simulink model "Simulink_Modell"  (R2017b)
settings: Solver=VariableStepAuto  StartTime=0.0  StopTime=10.0  RelTol=1e-3
libraries: simulink x3, aerolibatmos2 x1
settings Model: Creator=Christian Re  LastModifiedBy=Christian Re

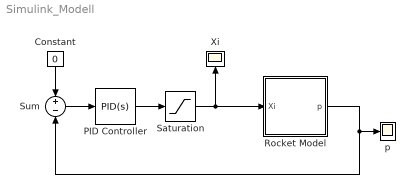
== system Simulink_Modell ==
  Constant : Constant  Value=0
  PID Controller : simulink/Continuous/PID Controller  Controller=PID  TimeDomain=Continuous-time  SampleTime=-1  IntegratorMethod=Forward Euler  FilterMethod=Forward Euler  Form=Parallel  UseFilter=on  ControllerParametersSource=internal  P=0.005  I=0.005  D=0.00008  N=100  InitialConditionSource=internal  InitialConditionForIntegrator=0  InitialConditionForFilter=0  ExternalReset=none  LimitOutput=off  UpperSaturationLimit=inf  LowerSaturationLimit=-inf  LinearizeAsGain=on  AntiWindupMode=none  Kb=1  TrackingMode=off  Kt=1  PParamMin=[]  PParamMax=[]  IParamMin=[]  IParamMax=[]  DParamMin=[]  DParamMax=[]  NParamMin=[]  NParamMax=[]  KbParamMin=[]  KbParamMax=[]  KtParamMin=[]  KtParamMax=[]  POutMin=[]  POutMax=[]  IOutMin=[]  IOutMax=[]  DOutMin=[]  DOutMax=[]  NOutMin=[]  NOutMax=[]  KbOutMin=[]  KbOutMax=[]  KtOutMin=[]  KtOutMax=[]  IntegratorOutMin=[]  IntegratorOutMax=[]  FilterOutMin=[]  FilterOutMax=[]  SumOutMin=[]  SumOutMax=[]  SumI1OutMin=[]  SumI1OutMax=[]  SumI2OutMin=[]  SumI2OutMax=[]  SumI3OutMin=[]  SumI3OutMax=[]  SumDOutMin=[]  SumDOutMax=[]  SaturationOutMin=[]  SaturationOutMax=[]  IntegratorContinuousStateAttributes=''  IntegratorStateMustResolveToSignalObject=off  IntegratorRTWStateStorageClass=Auto  FilterContinuousStateAttributes=''  FilterStateMustResolveToSignalObject=off  FilterRTWStateStorageClass=Auto  DifferentiatorICPrevScaledInput=0  DifferentiatorOutMin=[]  DifferentiatorOutMax=[]  InitialConditionSetting=State (most efficient)  FilterDiffOutCoefMin=[]  FilterDiffOutCoefMax=[]  SumDenOutMin=[]  SumDenOutMax=[]  SumNumOutMin=[]  SumNumOutMax=[]  ReciprocalOutMin=[]  ReciprocalOutMax=[]  DivideOutMin=[]  DivideOutMax=[]  TunerSelectOption=Frequency Response Based
  "Rocket Model " : Subsystem  TreatAsAtomicUnit=on
  Saturation : Saturate  UpperLimit=pi/4  LowerLimit=-pi/4
  Sum : Sum  Inputs=+-
  Xi : Scope
  p : Scope
  wires:
  Sum/1 -> PID Controller/1
  Constant/1 -> Sum/1
  "Rocket Model "/1(p) -> Sum/2, p/1
  PID Controller/1 -> Saturation/1
  Saturation/1 -> "Rocket Model "/1(Xi), Xi/1

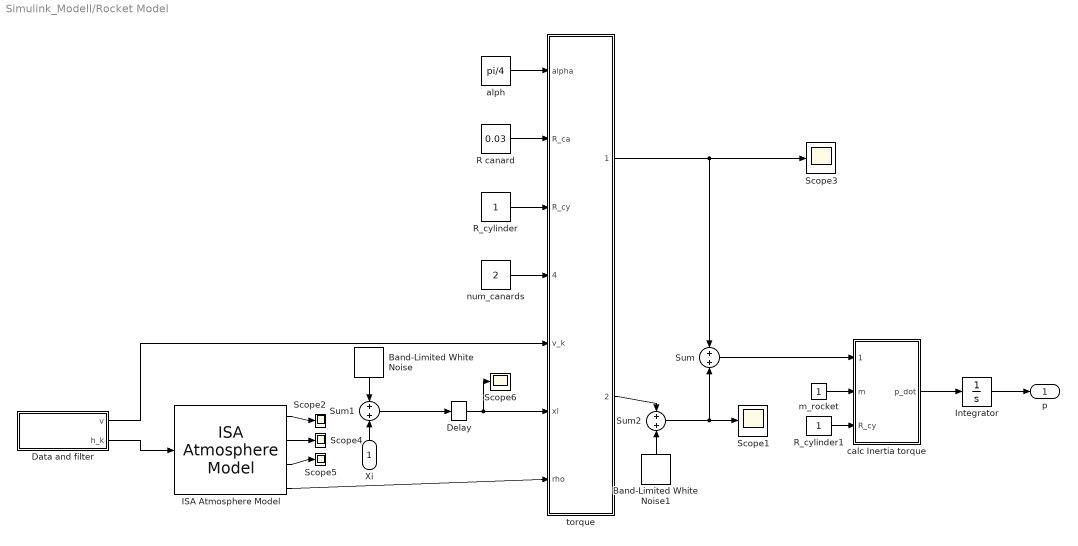
== system Simulink_Modell/Rocket Model  ==
  Xi : Inport
  Band-Limited White Noise : simulink/Sources/Band-Limited White Noise  Cov=[0.0000]  Ts=0.1  seed=[23341]
  Band-Limited White Noise1 : simulink/Sources/Band-Limited White Noise  Cov=[0.0]  Ts=0.1  seed=[23341]
  Data and filter : Subsystem  TreatAsAtomicUnit=on
  Delay : TransportDelay  DelayTime=0.00
  ISA Atmosphere Model : aerolibatmos2/ISA Atmosphere Model  custom=off  g=9.80665  gamma=1.4  R=287.0531  L=0.0065  h_trop=11000  h_strat=20000  rho0=1.225  P0=101325  T0=288.15  h0=0
      settings: SourceProductName=Aerospace Blockset
  Integrator : Integrator
  R canard : Constant  Value=0.03
  R_cylinder : Constant
  R_cylinder1 : Constant
  Scope{1..6} (6 alike) : Scope
  Sum : Sum
  Sum1 : Sum
  Sum2 : Sum
  "alph " : Constant  Value=pi/4
  calc Inertia torque : MATLAB Function  TreatAsAtomicUnit=on
  m_rocket : Constant
  "num_canards " : Constant  Value=2
  torque : MATLAB Function  TreatAsAtomicUnit=on
  p : Outport
  wires:
  "alph "/1 -> torque/1(alpha)
  R canard/1 -> torque/2(R_ca)
  Data and filter/1(v) -> torque/5(v_k)
  "num_canards "/1 -> torque/4(num_c)
  R_cylinder/1 -> torque/3(R_cy)
  m_rocket/1 -> calc Inertia torque/2(m)
  torque/1(M_canard) -> Scope3/1, Sum/1
  Sum/1 -> calc Inertia torque/1(M_sum)
  calc Inertia torque/1(p_dot) -> Integrator/1
  Integrator/1 -> p/1
  R_cylinder1/1 -> calc Inertia torque/3(R_cy)
  Band-Limited White Noise/1 -> Sum1/1
  Xi/1 -> Sum1/2
  Sum1/1 -> Delay/1
  Delay/1 -> Scope6/1, torque/6(xi)
  torque/2(M_disturb) -> Sum2/1
  Band-Limited White Noise1/1 -> Sum2/2
  Sum2/1 -> Scope1/1, Sum/2
  ISA Atmosphere Model/4 -> torque/7(rho)
  Data and filter/2(h_k) -> ISA Atmosphere Model/1
  ISA Atmosphere Model/3 -> Scope5/1
  ISA Atmosphere Model/2 -> Scope4/1
  ISA Atmosphere Model/1 -> Scope2/1

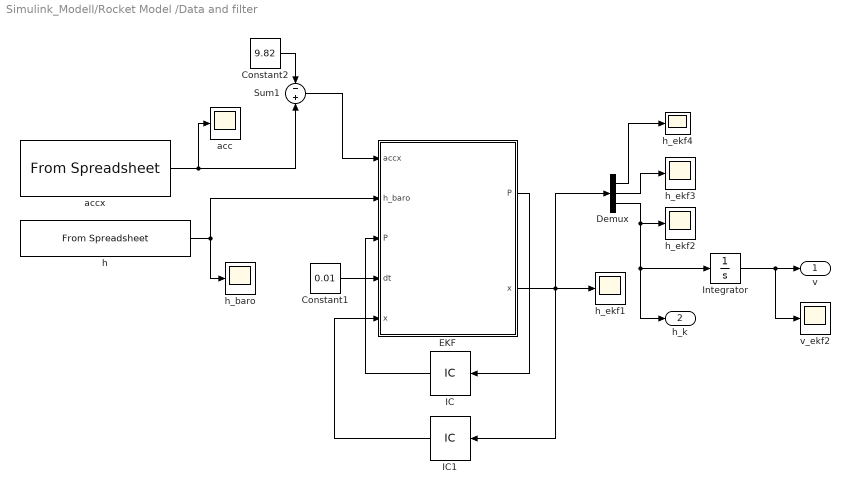
== system Simulink_Modell/Rocket Model /Data and filter ==
  Constant1 : Constant  Value=0.01
  Constant2 : Constant  Value=9.82
  Demux : Demux  Outputs=3
  EKF : MATLAB Function  TreatAsAtomicUnit=on
  IC : InitialCondition  Value=[0.0311 0.0491 0.0086 ;0.0491 0.1544 0.2023 ;0.0086 0.2023 4.5247]
  IC1 : InitialCondition  Value=[1.85 0.17/0.01 20]
  Integrator : Integrator
  Sum1 : Sum  Inputs=-+
  acc : Scope
  accx : FromSpreadsheet  FileName=C:\Users\Christian Re\Dropbox\HyEnD Electronics\Steuerung\Roll-Stabilization\Simulink-Modell\Data2.xlsx  SheetName=acc  Range=A2:B979
  h : FromSpreadsheet  FileName=C:\Users\Christian Re\Dropbox\HyEnD Electronics\Steuerung\Roll-Stabilization\Simulink-Modell\Data2.xlsx  SheetName=h  Range=A2:B979
  h_baro : Scope
  h_ekf{1..4} (4 alike) : Scope
  v_ekf2 : Scope
  v : Outport
  h_k : Outport  Port=2
  wires:
  Demux/3 -> Integrator/1, h_k/1, h_ekf2/1
  EKF/1(P) -> IC/1
  Demux/2 -> h_ekf3/1
  Constant1/1 -> EKF/4(dt)
  EKF/2(x) -> Demux/1, IC1/1, h_ekf1/1
  accx/1 -> acc/1, Sum1/2
  Sum1/1 -> EKF/1(accx)
  Constant2/1 -> Sum1/1
  Demux/1 -> h_ekf4/1
  Integrator/1 -> v/1, v_ekf2/1
  h/1 -> EKF/2(h_baro), h_baro/1
  IC1/1 -> EKF/5("x ")
  IC/1 -> EKF/3("P ")

== matlab function Simulink_Modell/Rocket Model /Data and filter/EKF ==
  data: P output; x output; accx input; h_baro input; P input; dt input; x input
function [P,x] = fcn(accx,h_baro,P,dt,x)
%% Initialize
sigma_baro= 1; %35.8229noise baro sensor;
sigma_acc= 5;%0.0002 %0.0012 noise acc sensor; 
z = [h_baro accx]; 
% a=0;
% v=0;
% h=0;
% x=[h;v;a]; %mean state vector %-------------
I = eye(3);
H= [1 0 0; 0 0 1];
F = [1 dt 1/2*dt^2; 0 1 dt; 0 0 1]; % StateTransitionFcn: maps previous state to next state
 
%P = [0.0311 0.0491 0.0086 ;0.0491 0.1544 0.2023 ;0.0086 0.2023 4.5247]; %needs change (loop)
% K = [0.0311 0.0003 ;0.0491 0.0081;0.0086 0.1810];%needs change (loop) unused

%% Measurement noise covariance matrix
% Autocovariance Least-Squares
% http://jbrwww.che.wisc.edu/software/als/

R= [sigma_baro^2 0; 0 sigma_acc^2]; % measurement noise covariance
Q = [0 0 0; 0 0 0; 0 0 1]; % process noise covariance matrix

%% Kalmanfilter
% Predict (marked as "1" in state)
x_n = F*x; %size(x_n) %+ B*u; %B*u:updated position due acc; B:control input matrix; u:control vector.
P_n=F*P*F'+Q; 
% Update (marked as "0" in state)
S= H*P_n*H'+R;
K =P_n*H'/S;
y= z'-H*x_n;	%size(y)    %trasposed because of array
x=x_n+K*y;          %size(x_n)
P=(I-K*H)*P_n;
end

== matlab function Simulink_Modell/Rocket Model /calc Inertia torque ==
  data: M_sum input; p_dot output; m input; R_cy input
function p_dot = fcn(M_sum,m,R_cy)
I = 0.5*m*R_cy^2; %inertia torque solid cylinder
p_dot = M_sum/I;

== matlab function Simulink_Modell/Rocket Model /torque ==
  data: alpha input; R_ca input; R_cy input; num_c input; v_k input; xi input; rho input; M_canard output; M_disturb output
function [M_canard,M_disturb] = fcn(alpha,R_ca,R_cy,num_c,v_k,xi,rho)
H = tan(alpha) * R_ca;
% fun_ca = @(r) (-H*r.^2/R_ca +H*r)*num_c/2*v_k^2*cos(xi)*sin(xi)*rho;
%fun_ca integrated: 

%M_canard=(H*(R_ca^3-3*R_ca*R_cy^2+2*R_cy^3)/(6*R_ca))*num_c/2*v_k^2*cos(xi)*sin(xi)*rho; % old%wrong 
 
M_canard = -num_c*rho*v_k^2*sin(xi)*sin(xi)*tan(alpha)*(R_ca^3-3*R_ca*R_cy^2+2*R_cy^3)/6; %new buggy

M_disturb =num_c*rho*v_k^2*sin(pi/16)*sin(pi/16)*tan(alpha)*(R_ca^3-3*R_ca*R_cy^2+2*R_cy^3)/6; %lift simulated by 2canards with pi/10 angle
